simulink model "nonlinear_Modell"  (R2023a)
settings: Solver=ode113  StartTime=0.0  StopTime=10  RelTol=1e-3
values from neighbouring files (symbols this model uses):
  A = []    [equilibrium.m]
  u_eq1 = double(u_eq1)    [linearModel.m]
  x_eq = [1 15 70]    [linearModel.m]
undefined symbols (not defined in the file or in its folder): B, C, uss
settings Model: Creator=derri  LastModifiedBy=derri

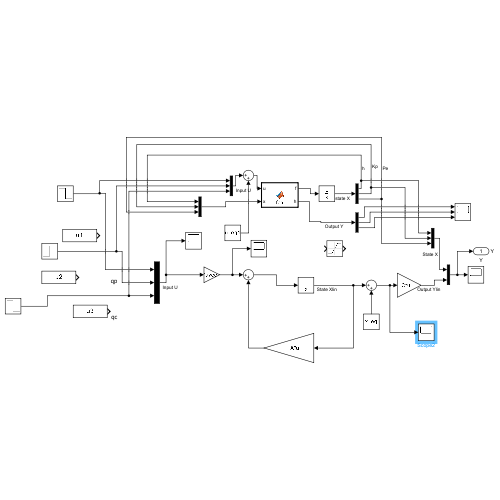
[thumbnail: Simulink's stored preview of the top-level diagram]
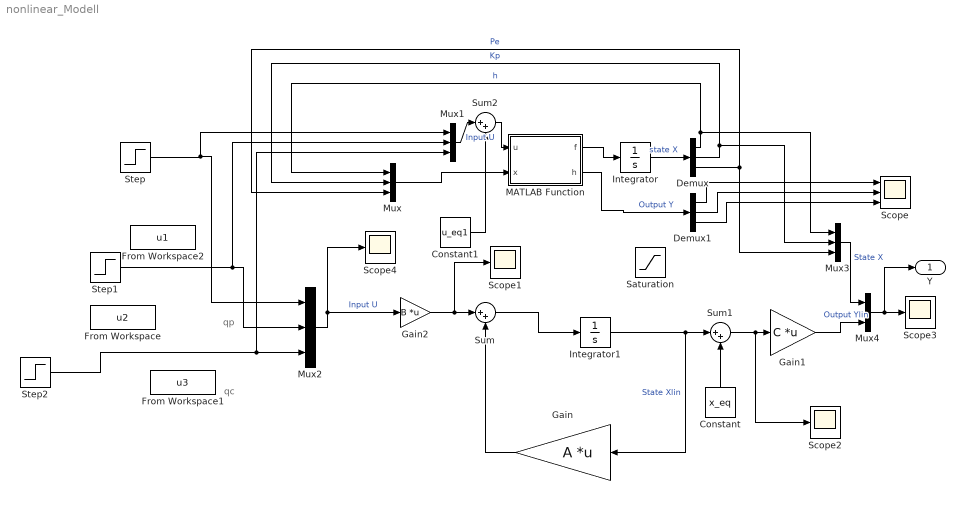
== system nonlinear_Modell ==
  note: qc
  note: qp
  Constant : Constant  Value=x_eq
  Constant1 : Constant  Value=u_eq1
  Demux : Demux  Outputs=3
  Demux1 : Demux  Outputs=3
  From Workspace : FromWorkspace  VariableName=u2
  From Workspace1 : FromWorkspace  VariableName=u3
  From Workspace2 : FromWorkspace  VariableName=u1
  Gain : Gain  Gain=A  Multiplication=Matrix(K*u)
  Gain1 : Gain  Gain=C  Multiplication=Matrix(K*u)
  Gain2 : Gain  Gain=B  Multiplication=Matrix(K*u) (u vector)
  Integrator : Integrator  InitialCondition=x_eq'
  Integrator1 : Integrator
  MATLAB Function : MATLAB Function  TreatAsAtomicUnit=on
  Mux{,1..3} (4 alike) : Mux  Inputs=3
  Mux4 : Mux  Inputs=2
  Saturation : Saturate
  Scope : Scope  NumInputPorts=3
  Scope{1..4} (4 alike) : Scope
  Step : Step  Time=0  After=uss(1)  SampleTime=0
  Step1 : Step  After=uss(2)  SampleTime=0
  Step2 : Step  Time=0  After=uss(3)  SampleTime=0
  Sum : Sum  Inputs=|++
  Sum1 : Sum  Inputs=|++
  Sum2 : Sum  Inputs=|++
  Y : Outport  SignalName=Y
  wires:
  Demux/1 -> Mux3/1, Mux/1  "h"
  Demux/2 -> Mux/2, Mux3/2  "Kp"
  Demux/3 -> Mux/3, Mux3/3  "Pe"
  Mux/1 -> MATLAB Function/2(x)
  Demux1/1 -> Scope/1
  Demux1/2 -> Scope/2
  Demux1/3 -> Scope/3
  MATLAB Function/2(h) -> Demux1/1  "Output Y"
  MATLAB Function/1(f) -> Integrator/1
  Sum/1 -> Integrator1/1
  Gain1/1 -> Mux4/2  "Output Ylin"
  Mux3/1 -> Mux4/1  "State X"
  Mux4/1 -> Y/1, Scope3/1
  Integrator/1 -> Demux/1  "state X"
  Gain2/1 -> Scope1/1, Sum/1
  Constant/1 -> Sum1/2
  Integrator1/1 -> Sum1/1, Gain/1  "State Xlin"
  Mux2/1 -> Gain2/1, Scope4/1  "Input U"
  Sum1/1 -> Gain1/1, Scope2/1
  Gain/1 -> Sum/2
  Step/1 -> Mux2/1, Mux1/1
  Step1/1 -> Mux1/2, Mux2/2
  Step2/1 -> Mux1/3, Mux2/3
  Constant1/1 -> Sum2/2
  Mux1/1 -> Sum2/1  "Input U"
  Sum2/1 -> MATLAB Function/1(u)

== matlab function nonlinear_Modell/MATLAB Function ==
  data: f output; h output; u input; x input
function [f,h] = fcn(u,x)
p=getparam_Gsp();
u1=u(1);
u2=u(2);
u3=u(3);
x1=x(1);
x2=x(2);
x3=x(3);
f=[p.a1*x3+p.a2*x2-p.b1*u1-p.b2*(u2+p.K*x1)-p.k1;...
-p.a3*x2*(u2+p.K*x1)+p.k2;...
-p.a4*x3-p.a5*x2+p.b3*u1-((p.a6*x3+p.b4)/(p.b5*u3+p.k3))*u3+p.k4
];
h=[x1; x2; x3];
